simulink model "P6_Simulink"  (R2023a)
settings: Solver=ode23  StartTime=0.0  StopTime=0.01  RelTol=1e-3
values from neighbouring files (symbols this model uses):
  C = 10e-6    (= 1e-05)    [P6_CD_CD.m]
  d = 0.4    [P6_CD_CD.m]
  L = 2e-3    (= 0.002)    [P6_CD_CD.m]
  R = 10    [P6_CD_CD.m]
settings Model: Creator=karen  LastModifiedBy=karen

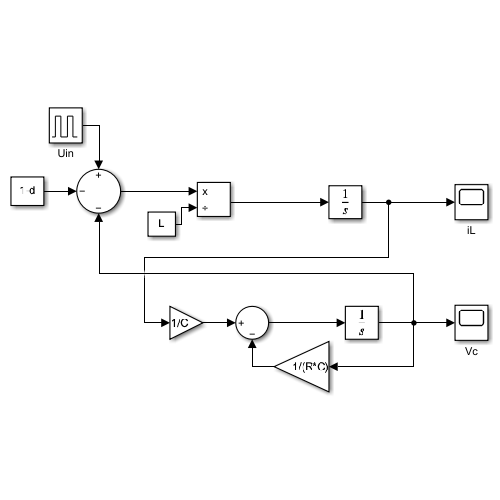
[thumbnail: Simulink's stored preview of the top-level diagram]
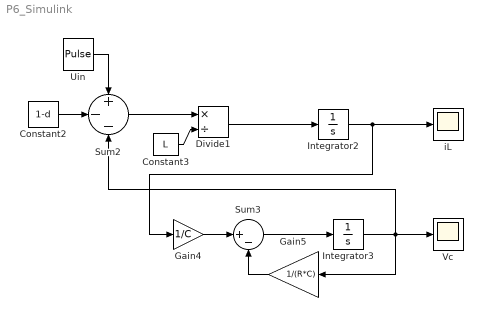
== system P6_Simulink ==
  Constant2 : Constant  Value=1-d
  Constant3 : Constant  Value=L
  Divide1 : Product  Inputs=*/
  Gain4 : Gain  Gain=1/C
  Gain5 : Gain  Gain=1/(R*C)
  Integrator2 : Integrator
  Integrator3 : Integrator
  Sum2 : Sum  Inputs=+--
  Sum3 : Sum  Inputs=|+-
  Uin : DiscretePulseGenerator  PulseType=Time based  Amplitude=32  Period=1e-5  PulseWidth=40
  Vc : Scope
  iL : Scope
  wires:
  Integrator2/1 -> Gain4/1, iL/1
  Divide1/1 -> Integrator2/1
  Sum2/1 -> Divide1/1
  Constant3/1 -> Divide1/2
  Sum3/1 -> Integrator3/1
  Gain4/1 -> Sum3/1
  Gain5/1 -> Sum3/2
  Integrator3/1 -> Vc/1, Sum2/3, Gain5/1
  Constant2/1 -> Sum2/2
  Uin/1 -> Sum2/1
